simulink model "s0502"  (Simulink 6.0)
settings: Solver=ode3  SolverMode=SingleTasking  StartTime=0.0  StopTime=900  FixedStep=1  MaxStep=1  RelTol=1e-3  AbsTol=1e-6
values from neighbouring files (symbols this model uses):
  wdach_ = wdach    (= 1)    [m0404Bsp.m]
  zdach_ = zdach    (= 1)    [m0404Bsp.m]
undefined symbols (not defined in the file or in its folder): nenStell, nenStoer, rnen, rzae, zaeStell, zaeStoer
settings Model: LastModifiedBy=Froriep
settings DataIOCC: LimitDataPoints=off  SaveOutput=off  SaveTime=off
settings OptimizationCC: BooleanDataType=off
settings DebuggingCC: SolverPrmCheckMsg=none
settings HardwareCC: TargetUnknown=on
settings STFCustomTargetCC: TargetFcnLib=ansi_tfl_tmw.mat  GenFloatMathFcnCalls=ANSI_C  ModelReferenceCompliant=off  SystemTargetFile=grt.tlc

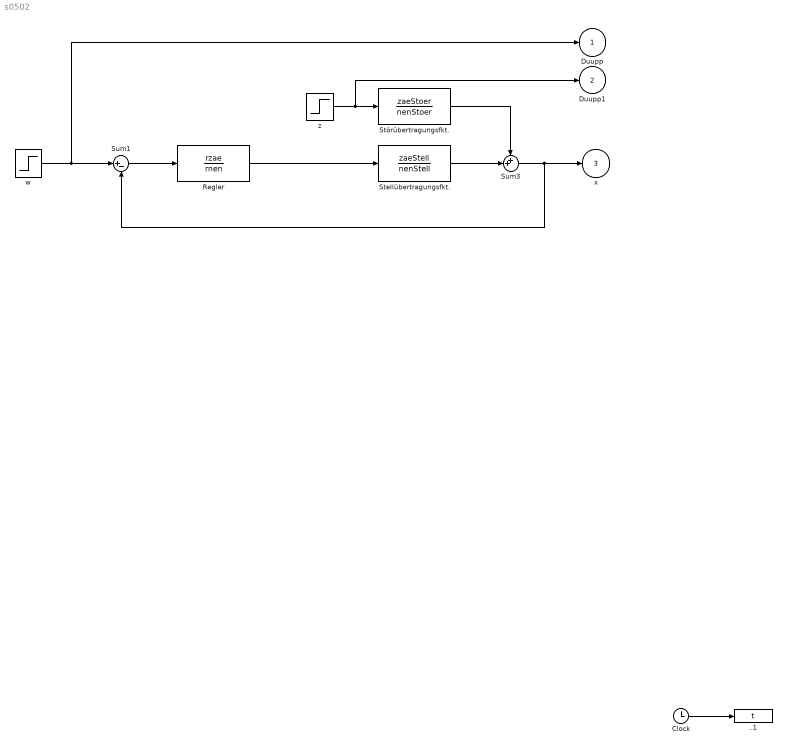
== system s0502 ==
  ..1 : ToWorkspace  VariableName=t  SaveFormat=Array
  Clock : Clock
      settings: Decimation=10
  Regler : TransferFcn  Numerator=rzae  Denominator=rnen
  Stellübertragungsfkt. : TransferFcn  Numerator=zaeStell  Denominator=nenStell
  Störübertragungsfkt. : TransferFcn  Numerator=zaeStoer  Denominator=nenStoer
  Sum1 : Sum  Inputs=|+-  SaturateOnIntegerOverflow=on  InputSameDT=on
  Sum3 : Sum  Inputs=++|  SaturateOnIntegerOverflow=on  InputSameDT=on
  w : Step  Time=0  After=wdach_  SampleTime=0
  z : Step  Time=0  After=zdach_  SampleTime=0
  Duupp : Outport
  Duupp1 : Outport  Port=2
  x : Outport  Port=3
  wires:
  z/1 -> Duupp1/1, Störübertragungsfkt./1
  w/1 -> Duupp/1, Sum1/1
  Sum1/1 -> Regler/1
  Clock/1 -> ..1/1
  Regler/1 -> Stellübertragungsfkt./1
  Stellübertragungsfkt./1 -> Sum3/2
  Störübertragungsfkt./1 -> Sum3/1
  Sum3/1 -> x/1, Sum1/2
